simulink model "ejemplo1"  (R2015a)
settings: Solver=ode45  StartTime=0.0  StopTime=10  RelTol=1e-3
libraries: simulink x1
settings Model: Creator=Amanda  LastModifiedBy=Amanda

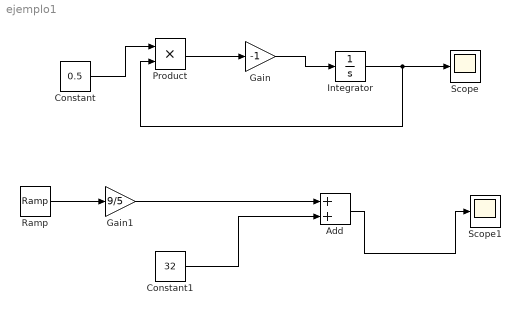
== system ejemplo1 ==
  Add : Sum
  Constant : Constant  Value=0.5
  Constant1 : Constant  Value=32
  Gain : Gain  Gain=-1
  Gain1 : Gain  Gain=9/5
  Integrator : Integrator  InitialCondition=5
  Product : Product
  Ramp : simulink/Sources/Ramp  slope=1  start=0  X0=0
  Scope : Scope
  Scope1 : Scope
      settings: TimeRange=10  YMin=95.609985  YMax=95.69190499999999
  wires:
  Constant/1 -> Product/1
  Product/1 -> Gain/1
  Gain/1 -> Integrator/1
  Integrator/1 -> Product/2, Scope/1
  Ramp/1 -> Gain1/1
  Gain1/1 -> Add/1
  Constant1/1 -> Add/2
  Add/1 -> Scope1/1
